simulink model "LLC_converter"  (R2024b)
settings: Solver=ode23tb  StartTime=0.0  StopTime=0.25  RelTol=1e-3
libraries: spsCurrentMeasurementLib x18, spsSeriesRLCBranchLib x15, spsDiodeLib x6, spsMosfetLib x6, spsVoltageMeasurementLib x6, spsDCVoltageSourceLib x3, spsLinearTransformerLib x3, spsMeanLib x3, spsTHDLib x3, sps_lib x1
settings Model: Creator=m_pek  LastModifiedBy=m_pek

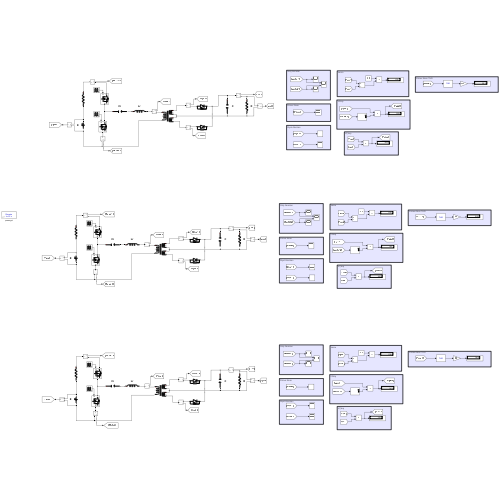
[thumbnail: Simulink's stored preview of the top-level diagram]
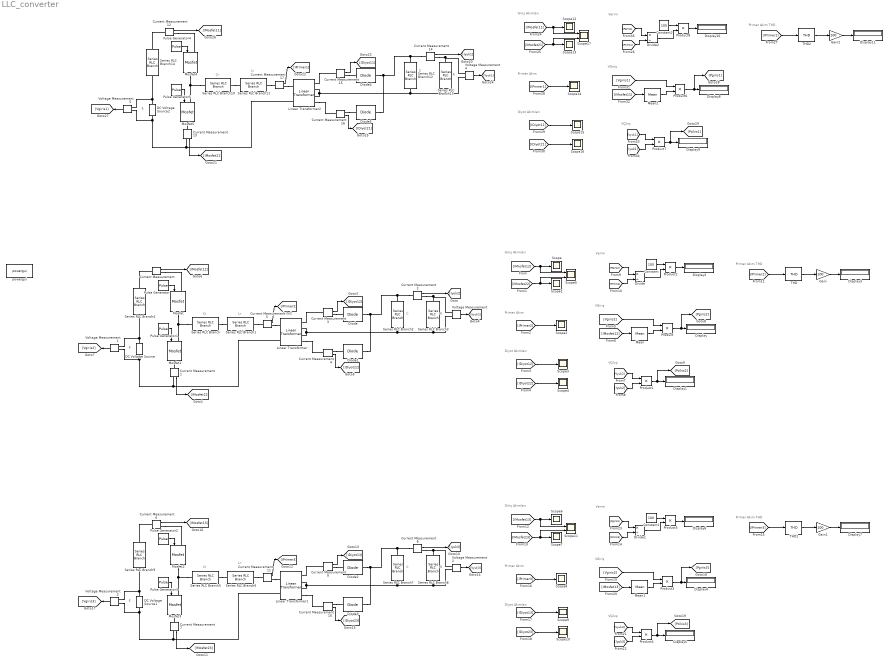
== system LLC_converter ==
  note: Verim
  note: Diyot Akımları
  note: Primer Akım THD
  note: VÇıkış
  note: VGiriş
  note: Primer Akım
  note: Giriş Akımları
  note: Cr
  note: Lr
  note: C
  note: R
  note: E
  note: Primer Akım THD
  note: VGiriş
  note: Diyot Akımları
  note: R
  note: Lr
  note: Cr
  note: E
  note: C
  note: VÇıkış
  note: Primer Akım
  note: Giriş Akımları
  note: Verim
  note: Primer Akım THD
  note: VGiriş
  note: Diyot Akımları
  note: R
  note: Lr
  note: Cr
  note: E
  note: C
  note: VÇıkış
  note: Primer Akım
  note: Giriş Akımları
  note: Verim
  Constant : Constant  Value=100
  Constant1 : Constant  Value=100
  Constant2 : Constant  Value=100
  Current Measurement{,1..17} (18 alike) : spsCurrentMeasurementLib/Current Measurement  PhasorSimulation=off  OutputType=Complex  PSBequivalent=0
  DC Voltage Source : spsDCVoltageSourceLib/DC Voltage Source  Amplitude=390  Measurements=None
  DC Voltage Source1 : spsDCVoltageSourceLib/DC Voltage Source  Amplitude=390  Measurements=None
  DC Voltage Source2 : spsDCVoltageSourceLib/DC Voltage Source  Amplitude=390  Measurements=None
  Diode{,1..5} (6 alike) : spsDiodeLib/Diode  Ron=0.001  Lon=0  Vf=0.8  IC=0  UseSnubber=0  Rs=500  Cs=250e-9  Measurements=off
  Display{,1..11} (12 alike) : Display
  Divide : Product  Inputs=*/
  Divide1 : Product  Inputs=*/
  Divide2 : Product  Inputs=*/
  Gain : Gain  Gain=100
  Gain1 : Gain  Gain=100
  Gain2 : Gain  Gain=100
  Linear Transformer : spsLinearTransformerLib/Linear Transformer  UNITS=SI  NominalPower=[ 300 150e3 ]  winding1=[36 0 0]  winding2=[4 0 0]  ThreeWindings=on  winding3=[4 0 0]  RmLm=[1e6 565e-06]  Measurements=None  DataType=on
  Linear Transformer1 : spsLinearTransformerLib/Linear Transformer  UNITS=SI  NominalPower=[ 300 150e3 ]  winding1=[36 0 0]  winding2=[4 0 0]  ThreeWindings=on  winding3=[4 0 0]  RmLm=[1e6 565e-06]  Measurements=None  DataType=on
  Linear Transformer2 : spsLinearTransformerLib/Linear Transformer  UNITS=SI  NominalPower=[ 300 150e3 ]  winding1=[36 0 0]  winding2=[4 0 0]  ThreeWindings=on  winding3=[4 0 0]  RmLm=[1e6 565e-06]  Measurements=None  DataType=on
  Mean : spsMeanLib/Mean  Freq=60  Vinit=0  Ts=0
  Mean1 : spsMeanLib/Mean  Freq=60  Vinit=0  Ts=0
  Mean2 : spsMeanLib/Mean  Freq=60  Vinit=0  Ts=0
  Mosfet{,1..5} (6 alike) : spsMosfetLib/Mosfet  Ron=0.1  Lon=0  Rd=0.01  Vfd=0  IC=0  Rs=1e5  Cs=inf  Measurements=off
  Product{,1..8} (9 alike) : Product
  Pulse Generator : DiscretePulseGenerator  PulseType=Time based  Period=1/100e3  PulseWidth=49
  Pulse Generator1 : DiscretePulseGenerator  PulseType=Time based  Period=1/100e3  PulseWidth=49  PhaseDelay=1/200e3
  Pulse Generator2 : DiscretePulseGenerator  PulseType=Time based  Period=1/130e3  PulseWidth=49
  Pulse Generator3 : DiscretePulseGenerator  PulseType=Time based  Period=1/130e3  PulseWidth=49  PhaseDelay=1/260e3
  Pulse Generator4 : DiscretePulseGenerator  PulseType=Time based  Period=1/70e3  PulseWidth=49
  Pulse Generator5 : DiscretePulseGenerator  PulseType=Time based  Period=1/70e3  PulseWidth=49  PhaseDelay=1/140e3
  Scope{,1..4,6..10,12..16} (15 alike) : Scope
  Scope11 : Scope  NumInputPorts=2
  Scope17 : Scope  NumInputPorts=2
  Scope5 : Scope  NumInputPorts=2
  Series RLC Branch : spsSeriesRLCBranchLib/Series RLC Branch  LConnTagsString=__new0  RConnTagsString=__new0  BranchType=C  Resistance=1  Inductance=1e-3  SetiL0=off  InitialCurrent=0  Capacitance=22e-9  Setx0=off  InitialVoltage=0  Measurements=None
  Series RLC Branch1 : spsSeriesRLCBranchLib/Series RLC Branch  LConnTagsString=__new0  RConnTagsString=__new0  BranchType=L  Resistance=1  Inductance=113e-6  SetiL0=off  InitialCurrent=0  Capacitance=1e-6  Setx0=off  InitialVoltage=0  Measurements=None
  Series RLC Branch10 : spsSeriesRLCBranchLib/Series RLC Branch  LConnTagsString=__new0  RConnTagsString=__new0  BranchType=C  Resistance=1  Inductance=1e-3  SetiL0=off  InitialCurrent=0  Capacitance=22e-9  Setx0=off  InitialVoltage=0  Measurements=None
  Series RLC Branch11 : spsSeriesRLCBranchLib/Series RLC Branch  LConnTagsString=__new0  RConnTagsString=__new0  BranchType=L  Resistance=1  Inductance=113e-6  SetiL0=off  InitialCurrent=0  Capacitance=1e-6  Setx0=off  InitialVoltage=0  Measurements=None
  Series RLC Branch12 : spsSeriesRLCBranchLib/Series RLC Branch  LConnTagsString=__new0  RConnTagsString=__new0  BranchType=C  Resistance=1  Inductance=1e-3  SetiL0=off  InitialCurrent=0  Capacitance=150e-3  Setx0=off  InitialVoltage=0  Measurements=None
  Series RLC Branch13 : spsSeriesRLCBranchLib/Series RLC Branch  LConnTagsString=__new0  RConnTagsString=__new0  BranchType=R  Resistance=2.4  Inductance=1e-3  SetiL0=off  InitialCurrent=0  Capacitance=1e-6  Setx0=off  InitialVoltage=0  Measurements=None
  Series RLC Branch14 : spsSeriesRLCBranchLib/Series RLC Branch  LConnTagsString=__new0  RConnTagsString=__new0  BranchType=R  Resistance=1e-6  Inductance=1e-3  SetiL0=off  InitialCurrent=0  Capacitance=1e-6  Setx0=off  InitialVoltage=0  Measurements=None
  Series RLC Branch2 : spsSeriesRLCBranchLib/Series RLC Branch  LConnTagsString=__new0  RConnTagsString=__new0  BranchType=C  Resistance=1  Inductance=1e-3  SetiL0=off  InitialCurrent=0  Capacitance=150e-3  Setx0=off  InitialVoltage=0  Measurements=None
  Series RLC Branch3 : spsSeriesRLCBranchLib/Series RLC Branch  LConnTagsString=__new0  RConnTagsString=__new0  BranchType=R  Resistance=2.4  Inductance=1e-3  SetiL0=off  InitialCurrent=0  Capacitance=1e-6  Setx0=off  InitialVoltage=0  Measurements=None
  Series RLC Branch4 : spsSeriesRLCBranchLib/Series RLC Branch  LConnTagsString=__new0  RConnTagsString=__new0  BranchType=R  Resistance=1e-6  Inductance=1e-3  SetiL0=off  InitialCurrent=0  Capacitance=1e-6  Setx0=off  InitialVoltage=0  Measurements=None
  Series RLC Branch5 : spsSeriesRLCBranchLib/Series RLC Branch  LConnTagsString=__new0  RConnTagsString=__new0  BranchType=C  Resistance=1  Inductance=1e-3  SetiL0=off  InitialCurrent=0  Capacitance=22e-9  Setx0=off  InitialVoltage=0  Measurements=None
  Series RLC Branch6 : spsSeriesRLCBranchLib/Series RLC Branch  LConnTagsString=__new0  RConnTagsString=__new0  BranchType=L  Resistance=1  Inductance=113e-6  SetiL0=off  InitialCurrent=0  Capacitance=1e-6  Setx0=off  InitialVoltage=0  Measurements=None
  Series RLC Branch7 : spsSeriesRLCBranchLib/Series RLC Branch  LConnTagsString=__new0  RConnTagsString=__new0  BranchType=C  Resistance=1  Inductance=1e-3  SetiL0=off  InitialCurrent=0  Capacitance=150e-3  Setx0=off  InitialVoltage=0  Measurements=None
  Series RLC Branch8 : spsSeriesRLCBranchLib/Series RLC Branch  LConnTagsString=__new0  RConnTagsString=__new0  BranchType=R  Resistance=2.4  Inductance=1e-3  SetiL0=off  InitialCurrent=0  Capacitance=1e-6  Setx0=off  InitialVoltage=0  Measurements=None
  Series RLC Branch9 : spsSeriesRLCBranchLib/Series RLC Branch  LConnTagsString=__new0  RConnTagsString=__new0  BranchType=R  Resistance=1e-6  Inductance=1e-3  SetiL0=off  InitialCurrent=0  Capacitance=1e-6  Setx0=off  InitialVoltage=0  Measurements=None
  THD : spsTHDLib/THD  Freq=100e3  Ts=0
  THD1 : spsTHDLib/THD  Freq=130e3  Ts=0
  THD2 : spsTHDLib/THD  Freq=70e3  Ts=0
  Voltage Measurement{,1..5} (6 alike) : spsVoltageMeasurementLib/Voltage Measurement  PhasorSimulation=off  OutputType=Complex  PSBequivalent=0
  powergui : sps_lib/powergui  Priority=1  SimulationMode=Discrete  SampleTime=1e-7  frequency=60  Iterations=50  frequencyindice=0  Pbase=100e6  ErrMax=1e-4  UnitsV=kV  UnitsW=MW  buscounter=0  FunctionMessages=off  echomessages=off  EnableUseOfTLC=off  CurrentSourceSwitches=off  DisableSnubberDevices=off  DisableRonSwitches=off  DisableVfSwitches=off  DisplayEquations=off  AutomaticDiscreteSolvers=off  SolverType=Tustin/Backward Euler (TBE)  Interpol=off  ExternalGateDelay=off  methode=off  Ts=100  x0status=blocks  SPID=on  SwTol=0  HookPort=off  NonlinearTolerance=1e-4  nMaxIteration=100  ContinueOnMaxIteration=off  RestoreLinks=warning  ResistiveCurrentMeasurement=off  Frange=[0:2:500]  Ylog=off  Xlog=on  ShowGrid=off  save=off  variable=ZData  structure=0  ZoomFFT=off  StartTime=0.0  cycles=1  DisplayStyle=1  fundamental=60  FreqAxis=off  MaxFrequency=1000  frequencyindicesteady=1  RmsSteady=1  display=off
  wires:
  Pulse Generator/1 -> Mosfet/1
  Pulse Generator1/1 -> Mosfet1/1
  Current Measurement/1 -> [IMosfet12]
  Current Measurement1/1 -> [IMosfet22]
  Current Measurement2/1 -> [Iyuk2]
  Current Measurement5/1 -> [IPrimer2]
  Current Measurement3/1 -> [IDiyot12]
  Voltage Measurement/1 -> [Vyuk2]
  Current Measurement4/1 -> [IDiyot22]
  Voltage Measurement1/1 -> [Vgiris2]
  [IMosfet12] -> Scope/1, Scope5/1
  [IMosfet22] -> Scope1/1, Scope5/2
  [IPrimer2] -> Scope2/1
  [IDiyot12] -> Scope3/1
  [IDiyot22] -> Scope4/1
  [Vgiris2] -> Product/1
  [Vyuk2] -> Product1/1
  [Iyuk2] -> Product1/2
  Product1/1 -> [Pcikis2], Display1/1
  [IMosfet12] -> Mean/1
  Mean/1 -> Product/2
  Product/1 -> [Pgiris2], Display/1
  [Pcikis2] -> Divide/2
  [Pgiris2] -> Divide/1
  Divide/1 -> Product2/2
  Constant/1 -> Product2/1
  Product2/1 -> Display2/1
  [IPrimer2] -> THD/1
  THD/1 -> Gain/1
  Gain/1 -> Display3/1
  [IDiyot13] -> Scope9/1
  Gain1/1 -> Display7/1
  [IDiyot23] -> Scope10/1
  [IMosfet23] -> Scope7/1, Scope11/2
  Product3/1 -> [Pgiris3], Display4/1
  [IMosfet13] -> Mean1/1
  Voltage Measurement2/1 -> [Vyuk3]
  Current Measurement9/1 -> [IDiyot13]
  Current Measurement6/1 -> [IMosfet13]
  Current Measurement11/1 -> [IPrimer3]
  Current Measurement8/1 -> [Iyuk3]
  [IMosfet13] -> Scope6/1, Scope11/1
  Mean1/1 -> Product3/2
  Constant1/1 -> Product5/1
  Current Measurement7/1 -> [IMosfet23]
  [Iyuk3] -> Product4/2
  [Vyuk3] -> Product4/1
  Voltage Measurement3/1 -> [Vgiris3]
  Product4/1 -> [Pcikis3], Display5/1
  Pulse Generator2/1 -> Mosfet2/1
  [IPrimer3] -> Scope8/1
  Product5/1 -> Display6/1
  THD1/1 -> Gain1/1
  Pulse Generator3/1 -> Mosfet3/1
  [Vgiris3] -> Product3/1
  Current Measurement10/1 -> [IDiyot23]
  [Pgiris3] -> Divide1/1
  [Pcikis3] -> Divide1/2
  [IPrimer3] -> THD1/1
  Divide1/1 -> Product5/2
  [IDiyot11] -> Scope15/1
  Gain2/1 -> Display11/1
  [IDiyot21] -> Scope16/1
  [IMosfet21] -> Scope13/1, Scope17/2
  Product6/1 -> [Pgiris1], Display8/1
  [IMosfet11] -> Mean2/1
  Voltage Measurement4/1 -> [Vyuk1]
  Current Measurement15/1 -> [IDiyot11]
  Current Measurement12/1 -> [IMosfet11]
  Current Measurement17/1 -> [IPrimer1]
  Current Measurement14/1 -> [Iyuk1]
  [IMosfet11] -> Scope12/1, Scope17/1
  Mean2/1 -> Product6/2
  Constant2/1 -> Product8/1
  Current Measurement13/1 -> [IMosfet21]
  [Iyuk1] -> Product7/2
  [Vyuk1] -> Product7/1
  Voltage Measurement5/1 -> [Vgiris1]
  Product7/1 -> [Pcikis1], Display9/1
  Pulse Generator4/1 -> Mosfet4/1
  [IPrimer1] -> Scope14/1
  Product8/1 -> Display10/1
  THD2/1 -> Gain2/1
  Pulse Generator5/1 -> Mosfet5/1
  [Vgiris1] -> Product6/1
  Current Measurement16/1 -> [IDiyot21]
  [Pgiris1] -> Divide2/1
  [Pcikis1] -> Divide2/2
  [IPrimer1] -> THD2/1
  Divide2/1 -> Product8/2
  connections:
  Current Measurement2/LConn1 -- Series RLC Branch2/LConn1 -- Diode1/RConn1 -- Diode/RConn1
  Series RLC Branch/LConn1 -- Mosfet1/LConn1 -- Mosfet/RConn1
  DC Voltage Source/LConn1 -- Current Measurement1/RConn1 -- Linear Transformer/LConn2 -- Voltage Measurement1/LConn2
  DC Voltage Source/RConn1 -- Series RLC Branch4/RConn1 -- Voltage Measurement1/LConn1
  Series RLC Branch/RConn1 -- Series RLC Branch1/LConn1
  Series RLC Branch1/RConn1 -- Current Measurement5/LConn1
  Linear Transformer/RConn1 -- Current Measurement3/LConn1
  Series RLC Branch3/RConn1 -- Linear Transformer/RConn2 -- Linear Transformer/RConn3 -- Series RLC Branch2/RConn1 -- Voltage Measurement/LConn2
  Linear Transformer/RConn4 -- Current Measurement4/LConn1
  Series RLC Branch4/LConn1 -- Current Measurement/LConn1
  Current Measurement/RConn1 -- Mosfet/LConn1
  Current Measurement1/LConn1 -- Mosfet1/RConn1
  Current Measurement2/RConn1 -- Voltage Measurement/LConn1 -- Series RLC Branch3/LConn1
  Current Measurement3/RConn1 -- Diode/LConn1
  Current Measurement4/RConn1 -- Diode1/LConn1
  Current Measurement5/RConn1 -- Linear Transformer/LConn1
  Current Measurement8/LConn1 -- Series RLC Branch7/LConn1 -- Diode3/RConn1 -- Diode2/RConn1
  DC Voltage Source1/RConn1 -- Series RLC Branch9/RConn1 -- Voltage Measurement3/LConn1
  Voltage Measurement2/LConn2 -- Linear Transformer1/RConn2 -- Linear Transformer1/RConn3 -- Series RLC Branch7/RConn1 -- Series RLC Branch8/RConn1
  Series RLC Branch8/LConn1 -- Current Measurement8/RConn1 -- Voltage Measurement2/LConn1
  Linear Transformer1/LConn2 -- Voltage Measurement3/LConn2 -- DC Voltage Source1/LConn1 -- Current Measurement7/RConn1
  Series RLC Branch5/LConn1 -- Mosfet3/LConn1 -- Mosfet2/RConn1
  Current Measurement10/RConn1 -- Diode3/LConn1
  Current Measurement7/LConn1 -- Mosfet3/RConn1
  Current Measurement9/RConn1 -- Diode2/LConn1
  Current Measurement11/RConn1 -- Linear Transformer1/LConn1
  Series RLC Branch6/RConn1 -- Current Measurement11/LConn1
  Series RLC Branch9/LConn1 -- Current Measurement6/LConn1
  Series RLC Branch5/RConn1 -- Series RLC Branch6/LConn1
  Linear Transformer1/RConn1 -- Current Measurement9/LConn1
  Linear Transformer1/RConn4 -- Current Measurement10/LConn1
  Current Measurement6/RConn1 -- Mosfet2/LConn1
  Current Measurement14/LConn1 -- Series RLC Branch12/LConn1 -- Diode5/RConn1 -- Diode4/RConn1
  DC Voltage Source2/RConn1 -- Series RLC Branch14/RConn1 -- Voltage Measurement5/LConn1
  Voltage Measurement4/LConn2 -- Linear Transformer2/RConn2 -- Linear Transformer2/RConn3 -- Series RLC Branch12/RConn1 -- Series RLC Branch13/RConn1
  Series RLC Branch13/LConn1 -- Current Measurement14/RConn1 -- Voltage Measurement4/LConn1
  Linear Transformer2/LConn2 -- Voltage Measurement5/LConn2 -- DC Voltage Source2/LConn1 -- Current Measurement13/RConn1
  Series RLC Branch10/LConn1 -- Mosfet5/LConn1 -- Mosfet4/RConn1
  Current Measurement16/RConn1 -- Diode5/LConn1
  Current Measurement13/LConn1 -- Mosfet5/RConn1
  Current Measurement15/RConn1 -- Diode4/LConn1
  Current Measurement17/RConn1 -- Linear Transformer2/LConn1
  Series RLC Branch11/RConn1 -- Current Measurement17/LConn1
  Series RLC Branch14/LConn1 -- Current Measurement12/LConn1
  Series RLC Branch10/RConn1 -- Series RLC Branch11/LConn1
  Current Measurement12/RConn1 -- Mosfet4/LConn1
  Linear Transformer2/RConn1 -- Current Measurement15/LConn1
  Linear Transformer2/RConn4 -- Current Measurement16/LConn1
